simulink model "sampleModel1789_1_sub_sub"  (R2023a)
settings: Solver=VariableStepAuto  StartTime=0.0  StopTime=10.0  RelTol=1e-3
libraries: hdlsllib x4, simulink x2
settings Model: Creator=user1  LastModifiedBy=user1

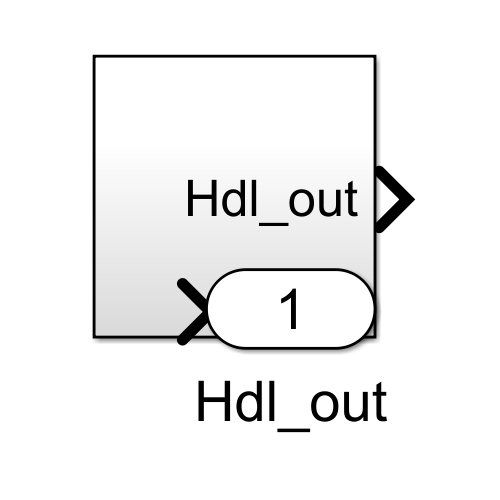
[thumbnail: Simulink's stored preview of the top-level diagram]
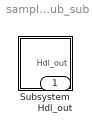
== system sampleModel1789_1_sub_sub ==
  Subsystem : Subsystem
  Hdl_out : Outport  OutDataTypeStr=uint8

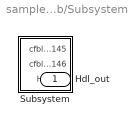
== system sampleModel1789_1_sub_sub/Subsystem ==
  Subsystem : Subsystem
  Hdl_out : Outport  OutDataTypeStr=uint8

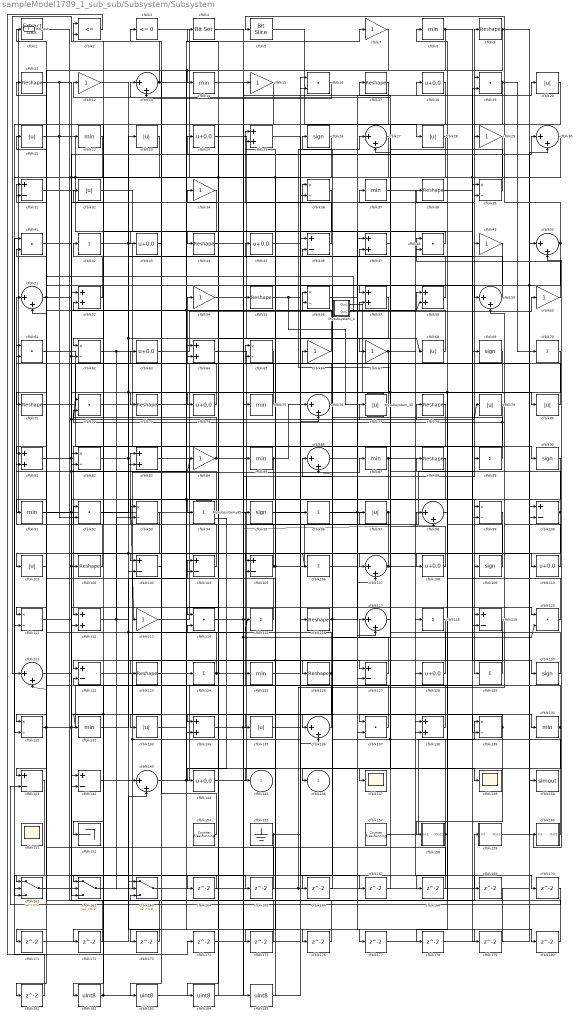
== system sampleModel1789_1_sub_sub/Subsystem/Subsystem ==
  Mysubsystem_35 : Subsystem  TreatAsAtomicUnit=on  RTWFcnName=Mysubsystem_35
      settings: RTWFcnNameOpts=User specified  RTWFileNameOpts=Use function name
  Mysubsystem_4 : Subsystem  TreatAsAtomicUnit=on  RTWFcnName=Mysubsystem_4
      settings: RTWFcnNameOpts=User specified  RTWFileNameOpts=Use function name
  Mysubsystem_45 : Subsystem  TreatAsAtomicUnit=on  RTWFcnName=Mysubsystem_45
      settings: RTWFcnNameOpts=User specified  RTWFileNameOpts=Use function name
  cfblk1 : simulink/Logic and Bit Operations/Extract Bits  bitsToExtract=Upper half  numBits=8  bitIdxRange=[0 7]  outScalingMode=Preserve fixed-point scaling
      settings: LibrarySourceBlock=|
      | hdlsllib/Logic and Bit
      | Operations/Extract Bits
  cfblk{31,46,100,103..105,119,122,127,141..142} (11 alike) : Sum  Inputs=+-  OutDataTypeStr=uint8
  cfblk{20..21,23,28,32,68,77,79..80,97,101,133,135} (13 alike) : Abs  OutDataTypeStr=uint8  SaturateOnIntegerOverflow=off
  cfblk{9,11,17,38,44,55,71,73,78,88,102,116,123,126} (14 alike) : Reshape
  cfblk{42,70,89,94,96,106,115,118,124,129} (10 alike) : Sum  Inputs=+  OutDataTypeStr=uint8
  cfblk{13,27,30,50..51,59,76,86,98,107,117,121,136,143} (14 alike) : Sum  Inputs=|++  OutDataTypeStr=uint8
  cfblk{18,24,43,45,63,74,108,110,128,144} (10 alike) : Bias  Bias=0.0  SaturateOnIntegerOverflow=off
  cfblk{26,69,90,95,109,130} (6 alike) : Signum
  cfblk{36,39,56,62,65,82,93,99,111,131,139} (11 alike) : Product  Inputs=*/  OutDataTypeStr=uint8  RndMeth=Zero  SaturateOnIntegerOverflow=on
  cfblk{25,47,52,57..58,64,81,83,112,134,138} (11 alike) : Sum  OutDataTypeStr=uint8
  cfblk{7,12,15,29,34,49,54,60,66..67,84,113} (12 alike) : Gain  OutDataTypeStr=uint8
  cfblk{16,19,41,48,61,72,92,114,120,137} (10 alike) : DotProduct  OutDataTypeStr=uint8
  cfblk{8,14,22,37,75,85,87,91,125,132,140} (11 alike) : MinMax  OutDataTypeStr=uint8
  cfblk147 : Scope
  cfblk149 : Scope
  cfblk150 : ToWorkspace  VariableName=simout  SaveFormat=Timeseries  SampleTime=-1
  cfblk151 : Scope
      settings: Floating=on
  cfblk152 : Terminator
  cfblk154 : hdlsllib/Sources/Counter Free-Running  NumBits=16  tsamp=-1
  cfblk155 : Ground
  cfblk157 : hdlsllib/Sources/Counter Free-Running  NumBits=16  tsamp=-1
  cfblk158 : Subsystem
      settings: LibrarySourceBlock=|
      | hdlsllib/Ports &
      | Subsystems/Subsystem
  cfblk159 : Subsystem
      settings: LibrarySourceBlock=|
      | hdlsllib/Ports &
      | Subsystems/Subsystem
  cfblk160 : Subsystem
      settings: LibrarySourceBlock=|
      | hdlsllib/Ports &
      | Subsystems/Subsystem
  cfblk161 : Switch  OutDataTypeStr=uint8  SaturateOnIntegerOverflow=off  InputSameDT=off
  cfblk162 : Switch  OutDataTypeStr=uint8  SaturateOnIntegerOverflow=off  InputSameDT=off
  cfblk163 : Switch  OutDataTypeStr=uint8  SaturateOnIntegerOverflow=off  InputSameDT=off
  cfblk{164..181} (18 alike) : Delay  SampleTime=1
  cfblk{182..185} (4 alike) : DataTypeConversion  OutDataTypeStr=uint8  SaturateOnIntegerOverflow=off  RndMeth=Floor
  cfblk2 : RelationalOperator  Operator=<=  OutDataTypeStr=boolean  InputSameDT=off
  cfblk3 : hdlsllib/Logic and Bit Operations/Compare To Zero  relop=<=  OutDataTypeStr=uint8
  cfblk4 : simulink/Logic and Bit Operations/Bit Set  iBit=0
      settings: LibrarySourceBlock=|
      | hdlsllib/Logic and Bit
      | Operations/Bit Set
  cfblk5 : hdlsllib/Logic and Bit Operations/Bit Slice  lidx=7  ridx=0
  cfblk145 : Outport  OutDataTypeStr=uint8  VectorParamsAs1DForOutWhenUnconnected=off
  cfblk146 : Outport  Port=2  OutDataTypeStr=uint8  VectorParamsAs1DForOutWhenUnconnected=off
  Hdl_out : Outport  Port=3  OutDataTypeStr=uint8
  wires:
  Mysubsystem_45/1(Out1) -> cfblk144/1
  Mysubsystem_4/2(Out2) -> cfblk91/1
  Mysubsystem_4/1(Out1) -> cfblk73/1
  cfblk185/1 -> cfblk105/2
  cfblk4/1 -> cfblk185/1
  cfblk184/1 -> cfblk4/1
  cfblk57/1 -> cfblk184/1
  cfblk183/1 -> cfblk15/1
  cfblk182/1 -> cfblk16/2, cfblk122/2
  cfblk181/1 -> cfblk41/1
  cfblk101/1 -> cfblk181/1
  cfblk180/1 -> cfblk82/1
  cfblk106/1 -> cfblk180/1
  cfblk179/1 -> cfblk48/2
  cfblk178/1 -> cfblk19/2
  cfblk177/1 -> cfblk50/1
  cfblk133/1 -> cfblk177/1
  cfblk176/1 -> cfblk163/1
  cfblk175/1 -> cfblk81/2
  cfblk174/1 -> cfblk16/1
  cfblk2/1 -> cfblk174/1
  cfblk173/1 -> cfblk52/1
  cfblk90/1 -> cfblk173/1
  cfblk172/1 -> cfblk142/1
  cfblk171/1 -> cfblk143/2
  cfblk170/1 -> cfblk141/2
  cfblk169/1 -> cfblk163/3
  cfblk168/1 -> cfblk114/2
  cfblk99/1 -> cfblk168/1
  cfblk167/1 -> cfblk117/1
  cfblk25/1 -> cfblk167/1
  cfblk166/1 -> cfblk86/1
  cfblk49/1 -> cfblk166/1
  cfblk165/1 -> cfblk1/1
  cfblk111/1 -> cfblk165/1
  cfblk164/1 -> cfblk161/2
  cfblk69/1 -> cfblk164/1
  cfblk59/1 -> cfblk47/2
  cfblk38/1 -> cfblk99/2
  cfblk125/1 -> cfblk139/2
  cfblk138/1 -> cfblk31/1
  cfblk87/1 -> cfblk112/2, cfblk170/1
  cfblk81/1 -> cfblk63/1, cfblk79/1, cfblk137/2
  cfblk129/1 -> cfblk65/2
  cfblk126/1 -> cfblk3/1, cfblk26/1, cfblk134/1
  cfblk7/1 -> cfblk14/1, cfblk103/1
  cfblk155/1 -> cfblk161/3, cfblk76/2
  cfblk92/1 -> cfblk23/1
  cfblk16/1 -> cfblk13/2
  cfblk37/1 -> cfblk110/1
  cfblk68/1 -> cfblk11/1
  cfblk17/1 -> cfblk111/2
  cfblk41/1 -> cfblk29/1
  cfblk115/1 -> cfblk21/1
  cfblk55/1 -> Mysubsystem_35/1(In1), cfblk19/1
  cfblk117/1 -> cfblk57/2
  cfblk29/1 -> cfblk81/1
  cfblk110/1 -> cfblk59/2
  cfblk11/1 -> cfblk92/2, cfblk22/1, cfblk102/1, cfblk119/1, cfblk36/2
  cfblk72/1 -> cfblk99/1
  cfblk83/1 -> cfblk138/1
  cfblk12/1 -> cfblk140/1, cfblk68/1
  cfblk154/1 -> cfblk13/1
  cfblk95/1 -> cfblk108/1
  cfblk96/1 -> cfblk47/1, cfblk109/1
  cfblk116/1 -> cfblk86/2, cfblk58/1
  cfblk71/1 -> cfblk30/2
  cfblk158/1(Out1) -> cfblk93/1, cfblk97/1, cfblk172/1
  cfblk19/1 -> cfblk132/1, cfblk152/1, cfblk70/1
  cfblk45/1 -> cfblk57/1
  cfblk5/1 -> cfblk28/1
  cfblk128/1 -> cfblk37/1
  cfblk94/1 -> cfblk61/2
  cfblk105/1 -> cfblk25/2, cfblk98/1, cfblk72/2
  cfblk44/1 -> cfblk20/1
  cfblk93/1 -> cfblk111/1
  cfblk109/1 -> cfblk24/1
  cfblk143/1 -> cfblk75/1, cfblk77/1
  cfblk161/1 -> cfblk62/2, cfblk36/1
  cfblk82/1 -> cfblk106/1, cfblk179/1, cfblk45/1
  cfblk22/1 -> cfblk131/2
  cfblk162/1 -> cfblk78/1
  cfblk123/1 -> cfblk7/1
  cfblk124/1 -> cfblk49/1, cfblk120/2, cfblk64/1, cfblk31/2
  cfblk61/1 -> cfblk124/1
  cfblk67/1 -> cfblk94/1, cfblk120/1
  cfblk130/1 -> cfblk92/1
  cfblk137/1 -> cfblk46/2
  cfblk60/1 -> cfblk48/1
  cfblk75/1 -> cfblk52/2
  cfblk132/1 -> cfblk104/1, cfblk115/1
  cfblk112/1 -> cfblk127/1, cfblk93/2
  cfblk56/1 -> cfblk107/2
  cfblk85/1 -> cfblk113/1, cfblk134/2, cfblk76/1
  cfblk73/1 -> cfblk30/1, cfblk58/2
  cfblk24/1 -> cfblk128/1
  cfblk66/1 -> cfblk32/1
  cfblk84/1 -> cfblk90/1, cfblk2/2
  cfblk120/1 -> cfblk8/1
  cfblk98/1 -> cfblk38/1
  cfblk135/1 -> cfblk116/1
  cfblk54/1 -> cfblk136/2
  cfblk36/1 -> cfblk62/1
  cfblk23/1 -> cfblk82/2
  cfblk8/1 -> cfblk130/1, cfblk104/2
  cfblk79/1 -> cfblk126/1
  cfblk100/1 -> cfblk27/2, cfblk127/2
  cfblk3/1 -> cfblk85/1
  cfblk70/1 -> cfblk147/1, cfblk162/3, cfblk178/1
  cfblk122/1 -> cfblk160/1(In1)
  cfblk121/1 -> cfblk56/2, cfblk84/1
  cfblk91/1 -> cfblk162/2, cfblk39/2
  cfblk48/1 -> cfblk44/1
  cfblk88/1 -> cfblk136/1
  cfblk139/1 -> cfblk137/1, cfblk158/1(In1)
  cfblk21/1 -> cfblk96/1, cfblk143/1
  cfblk27/1 -> cfblk135/1
  cfblk74/1 -> cfblk41/2
  cfblk134/1 -> cfblk39/1, cfblk98/2
  cfblk97/1 -> cfblk131/1, Hdl_out/1
  cfblk28/1 -> cfblk74/1, cfblk123/1
  cfblk20/1 -> cfblk114/1
  cfblk32/1 -> cfblk69/1
  cfblk77/1 -> cfblk34/1
  cfblk64/1 -> cfblk129/1
  cfblk89/1 -> cfblk61/1, cfblk72/1
  cfblk76/1 -> cfblk54/1
  cfblk9/1 -> cfblk150/1, cfblk141/1
  cfblk14/1 -> cfblk59/1
  cfblk127/1 -> cfblk56/1
  cfblk34/1 -> cfblk43/1
  cfblk113/1 -> cfblk65/1
  cfblk159/1(Out1) -> cfblk50/2
  cfblk15/1 -> cfblk182/1
  cfblk31/1 -> cfblk117/2
  cfblk86/1 -> cfblk18/1
  cfblk118/1 -> cfblk175/1, cfblk183/1
  cfblk30/1 -> cfblk145/1, cfblk51/2, cfblk119/2
  cfblk107/1 -> cfblk105/1, cfblk169/1
  cfblk160/1(Out1) -> cfblk125/1
  cfblk63/1 -> cfblk60/1
  cfblk58/1 -> cfblk2/1
  cfblk51/1 -> cfblk121/2, cfblk103/2
  cfblk43/1 -> cfblk133/1
  cfblk141/1 -> cfblk161/1
  cfblk47/1 -> cfblk107/1
  cfblk13/1 -> cfblk121/1, cfblk149/1
  cfblk39/1 -> cfblk12/1
  cfblk46/1 -> cfblk25/1
  cfblk157/1 -> cfblk139/1
  cfblk18/1 -> cfblk67/1
  cfblk50/1 -> cfblk100/2, cfblk71/1, cfblk5/1
  cfblk65/1 -> cfblk83/2, cfblk142/2
  cfblk26/1 -> cfblk101/1
  cfblk108/1 -> cfblk17/1
  cfblk42/1 -> cfblk118/1, cfblk176/1
  cfblk62/1 -> cfblk80/1, cfblk163/2
  cfblk114/1 -> cfblk9/1, cfblk89/1
  cfblk104/1 -> cfblk83/1
  cfblk136/1 -> cfblk95/1
  cfblk163/1 -> cfblk88/1, cfblk100/1
  cfblk78/1 -> cfblk112/1
  cfblk52/1 -> cfblk42/1
  cfblk131/1 -> cfblk46/1, cfblk138/2, cfblk171/1
  cfblk119/1 -> cfblk122/1
  cfblk102/1 -> cfblk51/1
  cfblk144/1 -> cfblk27/1
  cfblk1/1 -> cfblk159/1(In1)
  cfblk103/1 -> cfblk162/1
  cfblk140/1 -> cfblk146/1, cfblk64/2
  cfblk80/1 -> cfblk66/1
  cfblk142/1 -> cfblk87/1, cfblk55/1

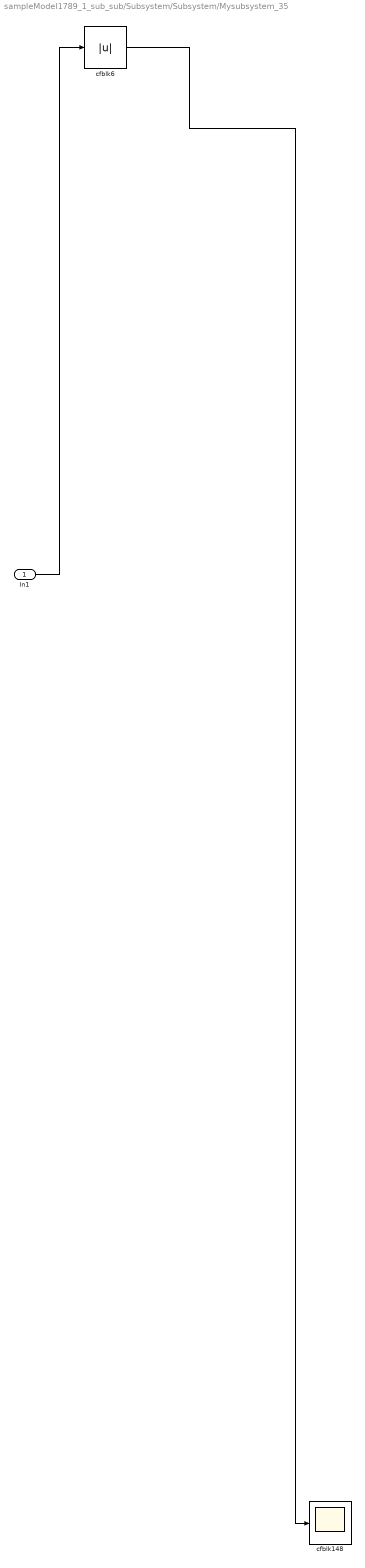
== system sampleModel1789_1_sub_sub/Subsystem/Subsystem/Mysubsystem_35 ==
  In1 : Inport
  cfblk148 : Scope
  cfblk6 : Abs  SaturateOnIntegerOverflow=off
  wires:
  cfblk6/1 -> cfblk148/1
  In1/1 -> cfblk6/1

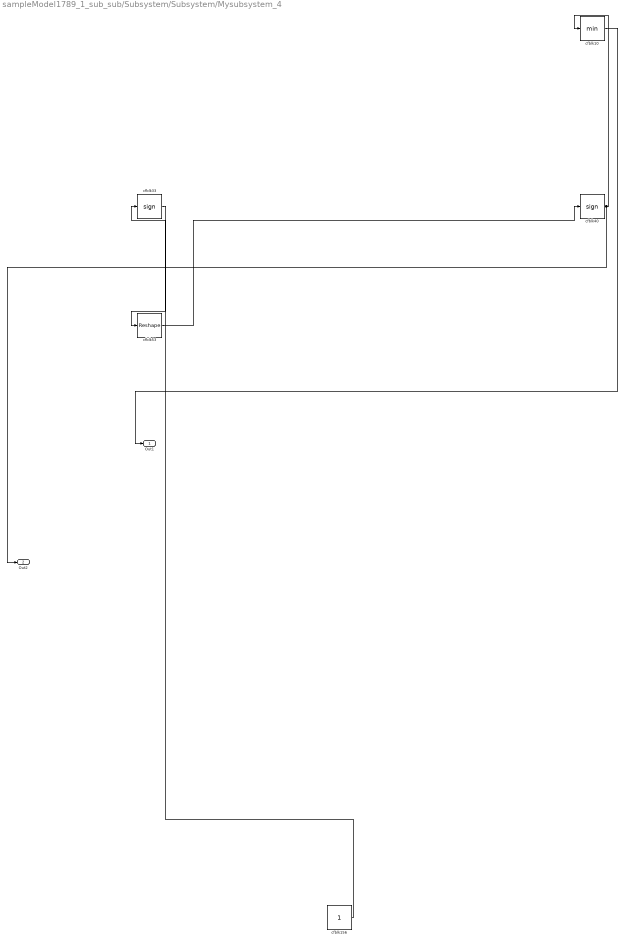
== system sampleModel1789_1_sub_sub/Subsystem/Subsystem/Mysubsystem_4 ==
  cfblk10 : MinMax
  cfblk156 : Constant  SampleTime=-1
  cfblk33 : Signum
  cfblk40 : Signum
  cfblk53 : Reshape
  Out1 : Outport
  Out2 : Outport  Port=2
  wires:
  cfblk53/1 -> cfblk40/1
  cfblk40/1 -> Out2/1, cfblk10/1
  cfblk10/1 -> Out1/1
  cfblk33/1 -> cfblk53/1
  cfblk156/1 -> cfblk33/1

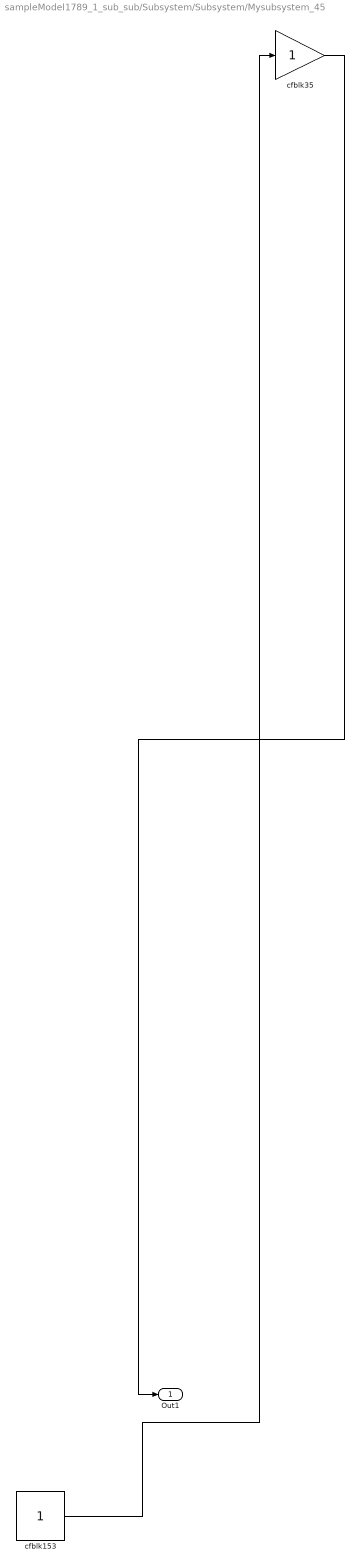
== system sampleModel1789_1_sub_sub/Subsystem/Subsystem/Mysubsystem_45 ==
  cfblk153 : Constant  SampleTime=-1
  cfblk35 : Gain
  Out1 : Outport
  wires:
  cfblk153/1 -> cfblk35/1
  cfblk35/1 -> Out1/1

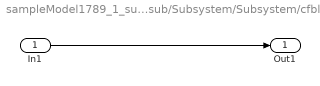
== system sampleModel1789_1_sub_sub/Subsystem/Subsystem/cfblk158 ==
  In1 : Inport
  Out1 : Outport
  wires:
  In1/1 -> Out1/1

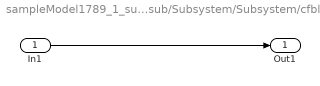
== system sampleModel1789_1_sub_sub/Subsystem/Subsystem/cfblk159 ==
  In1 : Inport
  Out1 : Outport
  wires:
  In1/1 -> Out1/1

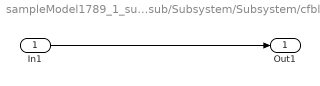
== system sampleModel1789_1_sub_sub/Subsystem/Subsystem/cfblk160 ==
  In1 : Inport
  Out1 : Outport
  wires:
  In1/1 -> Out1/1
